simulink subsystem "rss_spice_imported_mosfet_p_gate_charge_circuit"  (R2024a)
settings: Solver=VariableStepAuto  StartTime=0.0  StopTime=10.0  RelTol=1e-3
undefined symbols (not defined in the file): cstMoftExtRstn
libraries: fl_lib x7, nesl_utility x5, ee_lib x1
settings Model: Creator=pav2ofo  LastModifiedBy=pav2ofo

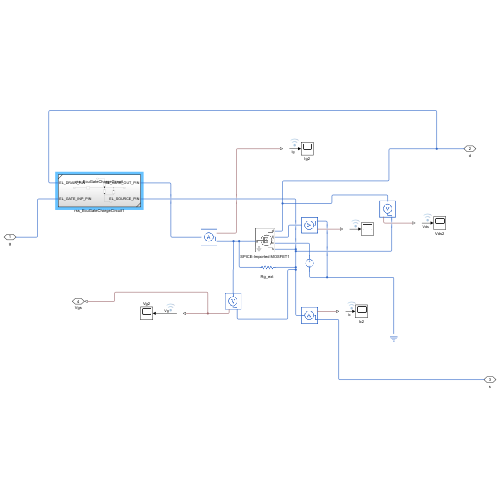
[thumbnail: Simulink's stored preview of the top-level diagram]
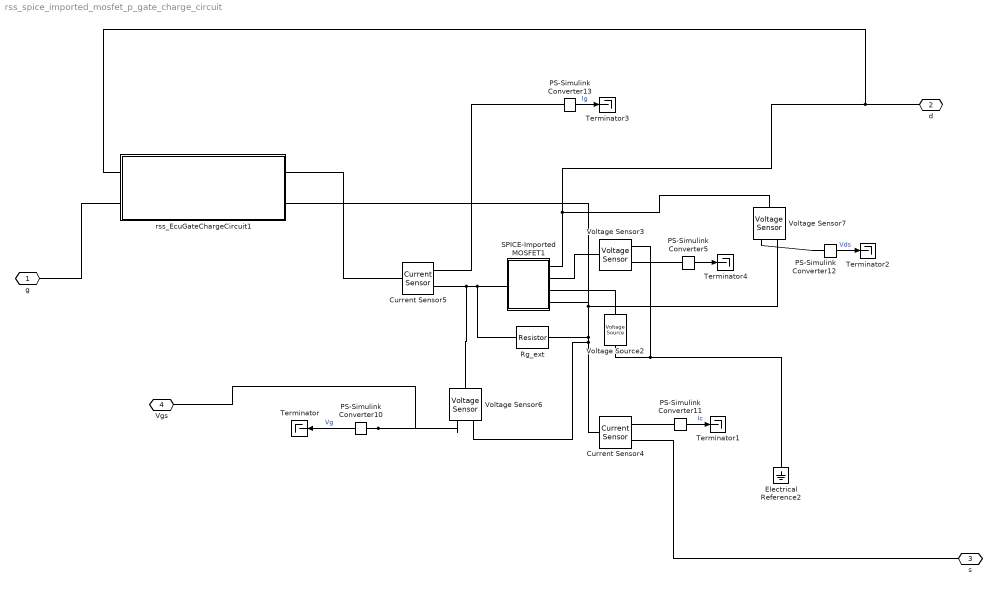
== system rss_spice_imported_mosfet_p_gate_charge_circuit ==
  Current Sensor4 : fl_lib/Electrical/Electrical Sensors/Current Sensor
  Current Sensor5 : fl_lib/Electrical/Electrical Sensors/Current Sensor
  Electrical Reference2 : fl_lib/Electrical/Electrical Elements/Electrical Reference
  PS-Simulink Converter{5,10..13} (5 alike) : nesl_utility/PS-Simulink Converter  PhysicalDomain=network_engine_domain  SubClassName=ps_output  LeftPortType=input  RightPortType=output  PseudoPeriodic=off  Frequencies=[]  VectorFormat=inherit  Unit=inherit  AffineConversion=off
  Rg_ext : fl_lib/Electrical/Electrical Elements/Resistor  R=cstMoftExtRstn kOhm  i_specify=off  i_priority=None  i=0 A  i_nominal_specify=off  i_nominal_value=1  i_nominal_unit=A  v_specify=off  v_priority=None  v=0 V  v_nominal_specify=off  v_nominal_value=1  v_nominal_unit=V
  SPICE-Imported MOSFET1 : Subsystem  mask(SPICE-Imported MOSFET){SeriesChoice=Infineon OptiMOS6 40V, DeviceOptiMOS40V=IAUC100N04S6N022, DeviceOptiMOS60V=IPB120N06S4_H1, DeviceOptiMOS80V=IAUT300N08S5N012, DeviceOptiMOS120V=IPB100N12S3_05}
      mask prompts: SeriesChoice "Series"; DeviceOptiMOS40V "Device"; DeviceOptiMOS60V "Device"; DeviceOptiMOS80V "Device"; DeviceOptiMOS120V "Device"
      mask help: MOSFET model converted from SPICE.<br/> <br/> To view information pertaining to this device model, see the <a href="matlab: ee.internal.spice.openAndGoToLine('Infineon-OptiMOS6_40V-SimulationModels-v02_00-EN.lib','IAUC100N04S6N022')">originating SPICE file</a>.
      mask init:
      | ee.internal.spice.maskCallbackMOSFETs(gcb)
      settings: CopyFcn=set_param(gcb,'LinkStatus','none');
      mask Help: web([docroot '/physmod/sps/ref/spiceimportedmosfet.html'])
      mask TypeOptions SeriesChoice: Infineon OptiMOS6 40V | Infineon OptiMOS4 60V | Infineon OptiMOS5 80V | Infineon OptiMOST 120V
      mask Callback SeriesChoice:
      | %Run mask initialization to update the block help
      | ee.internal.spice.maskCallbackMOSFETs(gcb)
      mask TypeOptions DeviceOptiMOS40V: IAUC120N04S6N009 | IAUC120N04S6N010 | IAUC120N04S6N013 | IAUC100N04S6N015 | IAUC100N04S6N022 | IAUC100N04S6N028 | IAUC80N04S6N036 | IAUC60N04S6N044 | IAUC120N04S6L008 | IAUC120N04S6L009 | IAUC120N04S6L012 | IAUC100N04S6L014 | IAUC100N04S6L020 | IAUC100N04S6L025 | IAUC80N04S6L032 | IAUC60N04S6L039
      mask Callback DeviceOptiMOS40V:
      | %Run mask initialization to update the block help
      | ee.internal.spice.maskCallbackMOSFETs(gcb)
      mask TypeOptions DeviceOptiMOS60V: IPB180N06S4_H1 | IPB120N06S4_H1 | IPI120N06S4_H1 | IPP120N06S4_H1 | IPB120N06S4_02 | IPI120N06S4_02 | IPP120N06S4_02 | IPB120N06S4_03 | IPI120N06S4_03 | IPP120N06S4_03 | IPB90N06S4_04 | IPD90N06S4_04 | IPD100N06S4_03 | IPI90N06S4_04 | IPP90N06S4_04 | IPB80N06S4_05 | IPD90N06S4_05 | IPI80N06S4_05 | IPP80N06S4_05 | IPB80N06S4_07 | IPD90N06S4_07 | IPI80N06S4_07 | IPP80N06S4_07 | IPB45N06S4_09 | IPD50N06S4_09 | IPI45N06S4_09 | IPP45N06S4_09 | IPG20N06S4_15 | IPB90N06S4L_04 | IPD90N06S4L_03 | IPI90N06S4L_04 | IPP90N06S4L_04 | IPB80N06S4L_05 | IPD90N06S4L_05 | IPI80N06S4L_05 | IPP80N06S4L_05 | IPB80N06S4L_07 | IPD90N06S4L_06 | IPI80N06S4L_07 | IPP80N06S4L_07 | IPB45N06S4L_08 | IPD50N06S4L_08 | IPI45N06S4L_08 | IPP45N06S4L_08 | IPD50N06S4L_12 | IPD30N06S4L_23 | IPD25N06S4L_30 | IPG20N06S4L_11 | IPG20N06S4L_14 | IPG20N06S4L_26
      mask Callback DeviceOptiMOS60V:
      | %Run mask initialization to update the block help
      | ee.internal.spice.maskCallbackMOSFETs(gcb)
      mask TypeOptions DeviceOptiMOS80V: IPB015N08N5 | IPB017N08N5 | IPP020N08N5 | IPT012N08N5 | IPB020N08N5 | IPP023N08N5 | IPB024N08N5 | IPP027N08N5 | IPB031N08N5 | IPP034N08N5 | IPB049N08N5 | IPP052N08N5 | IAUT300N08S5N012 | IAUT165N08S5N029 | IAUT300N08S5N014 | IAUT240N08S5N019 | IAUT200N08S5N023 | IAUS300N08S5N013T | IAUS300N08S5N015T | IAUC100N08S5N031 | IAUC100N08S5N043 | IAUC70N08S5N074
      mask Callback DeviceOptiMOS80V:
      | %Run mask initialization to update the block help
      | ee.internal.spice.maskCallbackMOSFETs(gcb)
      mask TypeOptions DeviceOptiMOS120V: IPB100N12S3_05 | IPI100N12S3_05 | IPP100N12S3_05 | IPB70N12S3_11 | IPI70N12S3_11 | IPP70N12S3_11 | IPD70N12S3_11 | IPD70N12S3L_12 | IPB70N12S3L_12 | IPI70N12S3L_12 | IPP70N12S3L_12 | IPB50N12S3L_15 | IPD50N12S3L_15 | IPI50N12S3L_15 | IPP50N12S3L_15 | IPB35N12S3L_26 | IPD35N12S3L_24 | IPD30N12S3L_31
      mask Callback DeviceOptiMOS120V:
      | %Run mask initialization to update the block help
      | ee.internal.spice.maskCallbackMOSFETs(gcb)
      mask DialogControl ParameterGroupVar Prompt: Device selection
  Terminator{,1..4} (5 alike) : Terminator
  Voltage Sensor3 : fl_lib/Electrical/Electrical Sensors/Voltage Sensor
  Voltage Sensor6 : fl_lib/Electrical/Electrical Sensors/Voltage Sensor
  Voltage Sensor7 : fl_lib/Electrical/Electrical Sensors/Voltage Sensor
  Voltage Source2 : ee_lib/Sources/Voltage Source  dc_voltage=25 V  ac_voltage=0 V  ac_shift=0 rad  ac_frequency=60 Hz  noise_mode=ee.enum.sources.noise.Disabled  PSD=0 V^2/Hz  sample_time=1e-3 s  repeatability=ee.enum.sources.repeatability.NotRepeatable  user_seed=0  auto_seed=3530215255  i_specify=off  i_priority=None  i=0 A  i_nominal_specify=off  i_nominal_value=1  i_nominal_unit=A  v_specify=off  v_priority=None  v=0 V  v_nominal_specify=off  v_nominal_value=1  v_nominal_unit=V
  rss_EcuGateChargeCircuit1 : Subsystem  ReferencedSubsystem=rss_EcuGateChargeCircuit
  g : PMIOPort  Side=Left
  d : PMIOPort  Port=2  Side=Right
  s : PMIOPort  Port=3  Side=Right
  Vgs : PMIOPort  Port=4  Side=Left
  wires:
  PS-Simulink Converter11/1 -> Terminator1/1  "Ic"
  PS-Simulink Converter10/1 -> Terminator/1  "Vg"
  PS-Simulink Converter5/1 -> Terminator4/1
  PS-Simulink Converter12/1 -> Terminator2/1  "Vds"
  PS-Simulink Converter13/1 -> Terminator3/1  "Ig"
  connections:
  Voltage Sensor6/RConn2 -- SPICE-Imported MOSFET1/RConn4 -- rss_EcuGateChargeCircuit1/RConn2 -- Voltage Sensor7/RConn2 -- Rg_ext/RConn1 -- Current Sensor4/LConn1
  rss_EcuGateChargeCircuit1/LConn1 -- SPICE-Imported MOSFET1/RConn1 -- Voltage Sensor7/LConn1 -- d/RConn1
  Voltage Sensor6/LConn1 -- SPICE-Imported MOSFET1/LConn1 -- Rg_ext/LConn1 -- Current Sensor5/RConn2
  Electrical Reference2/LConn1 -- Voltage Source2/RConn1 -- Voltage Sensor3/RConn2
  PS-Simulink Converter10/LConn1 -- Vgs/RConn1 -- Voltage Sensor6/RConn1
  g/RConn1 -- rss_EcuGateChargeCircuit1/LConn2
  SPICE-Imported MOSFET1/RConn3 -- Voltage Source2/LConn1
  rss_EcuGateChargeCircuit1/RConn1 -- Current Sensor5/LConn1
  Current Sensor4/RConn1 -- PS-Simulink Converter11/LConn1
  PS-Simulink Converter12/LConn1 -- Voltage Sensor7/RConn1
  Current Sensor5/RConn1 -- PS-Simulink Converter13/LConn1
  Current Sensor4/RConn2 -- s/RConn1
  Voltage Sensor3/RConn1 -- PS-Simulink Converter5/LConn1
  SPICE-Imported MOSFET1/RConn2 -- Voltage Sensor3/LConn1

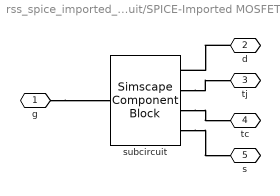
== system rss_spice_imported_mosfet_p_gate_charge_circuit/SPICE-Imported MOSFET1 ==
  subcircuit : SimscapeComponentBlock  SourceFile=ee_spice_mosfets.spiceinfineon.spiceOptiMOS_6_40V.IAUC100N04S6N022_wrapped  ComponentPath=ee_spice_mosfets.spiceinfineon.spiceOptiMOS_6_40V.IAUC100N04S6N022_wrapped  ComponentVariants="[\"ee_spice_mosfets.spiceinfineon.spiceOptiMOS_6_40V.IAUC100N04S6N022_wrapped\"]"  ComponentVariantNames="[\"IAUC100N04S6N022_wrapped\"]"  ClassName=IAUC100N04S6N022_wrapped  SchemaVersion=1
      settings: CopyFcn=simscape.engine.sli.internal.componentblockcallback(gcbh,'COPY')  PreCopyFcn=simscape.engine.sli.internal.componentblockcallback(gcbh,'PRECOPY')  PreDeleteFcn=simscape.engine.sli.internal.componentblockcallback(gcbh,'PREDELETE')  InternalSimscapePortConfiguration="{\"Bottom\":[],\"Left\":[{\"id\":\"gate\",\"label\":\"g\",\"type\":\"foundation.electrical.electrical\"}],\"Right\":[{\"id\":\"drain\",\"label\":\"d\",\"type\":\"foundation.electrical.electrical\"},{\"id\":\"tj\",\"label\":\"tj\",\"type\":\"foundation.electrical.electrical\"},{\"id\":\"tcase\",\"label\":\"tc\",\"type\":\"foundation.electrical.electrical\"},{\"id\":\"source\",\"label\":\"s\",\"type\":\"foundation.electrical.electrical\"}],\"Top\":[]}"
      mask Type: Infineon IAUC100N04S6N022
  g : PMIOPort  Side=Left
  d : PMIOPort  Port=2  Side=Right
  tj : PMIOPort  Port=3  Side=Right
  tc : PMIOPort  Port=4  Side=Right
  s : PMIOPort  Port=5  Side=Right
  connections:
  g/RConn1 -- subcircuit/LConn1
  d/RConn1 -- subcircuit/RConn1
  subcircuit/RConn2 -- tj/RConn1
  subcircuit/RConn3 -- tc/RConn1
  subcircuit/RConn4 -- s/RConn1
